simulink model "FMReceiverSimulinkExample"  (R2022b)
settings: Solver=FixedStepDiscrete  StartTime=0.0  StopTime=inf  RelTol=1e-3
PreLoadFcn:
  | fmRxParams = helperFMConfig;
PostLoadFcn:
  | rxBlock = find_system(gcs, 'MaskType', 'SDRu Receiver');
  | if exist('sdruroot', 'file')
  |     setupsdru;
  |     connectedRadios = findsdru;
  |     if strncmp(connectedRadios(1).Status, 'Success', 7)
  |         platform = connectedRadios(1).Platform;
  |         set_param(rxBlock{1}, 'Platform', platform);
  |         switch connectedRadios(1).Platform
  |             case {'B200','B210'}
  |                 address = connectedRadios(1).SerialNum;
  |                 fmRxParams.MasterClockRate = 20e6;
  |                 fmRxParams.DecimationFactor = (fmRxParams.MasterClockRate)/200e3;
  | %                 set_param(rxBlock{1}, 'masterClkRateB210', 'fmRxParams.MasterClockRate');
  | %                 set_param(rxBlock{1}, 'masterClkRateB200', 'fmRxParams.MasterClockRate');
  | %                 set_param(rxBlock{1}, 'decimInterp', 'fmRxParams.DecimationFactor');
  |             case {'X300','X310','N320/N321'}
  |                 address = connectedRadios(1).IPAddress;
  |                 fmRxParams.MasterClockRate = 200e6;
  |                 fmRxParams.DecimationFactor = (fmRxParams.MasterClockRate)/200e3;
  |             case {'N300','N310'}
  |                 address = connectedRadios(1).IPAddress;
  |                 fmRxParams.MasterClockRate = 153.6e6;
  |                 fmRxParams.DecimationFactor = (fmRxParams.MasterClockRate)/200e3;
  |             case {'N200/N210/USRP2'}
  |                 address = connectedRadios(1).IPAddress;
  |                 fmRxParams.MasterClockRate = 100e6;
  |                 fmRxParams.DecimationFactor = (fmRxParams.MasterClockRate)/200e3;
  |         end
  |     else
  |         platform = 'N200/N210/USRP2';
  |         address = '192.168.10.2';
  |         set_param(rxBlock{1}, 'Platform', platform);
  |         fmRxParams.MasterClockRate = 100e6;
  |         fmRxParams.DecimationFactor = (fmRxParams.MasterClockRate)/200e3;
  |     end
  |     set_param(rxBlock{1}, 'USRP_ID', address);
  | end
InitFcn:
  | fmRxParams = helperFMConfig;
  | 
  | if (strcmp(get_param([gcs '/Signal Source Selector'],'OverrideUsingVariant'),'V_4'))
  | rxBlock = find_system(gcs, 'MaskType', 'SDRu Receiver');
  | platform = get_param(rxBlock{1}, 'platform');
  | 
  | switch platform
  |     case {'B200','B210'}
  |         fmRxParams.MasterClockRate = 20e6;
  |         fmRxParams.DecimationFactor = (fmRxParams.MasterClockRate)/200e3;
  |     case {'X300','X310','N320/N321'}
  |         fmRxParams.MasterClockRate = 200e6;
  |         fmRxParams.DecimationFactor = (fmRxParams.MasterClockRate)/200e3;
  |     case {'N300','N310'}
  |         fmRxParams.MasterClockRate = 153.6e6;
  |         fmRxParams.DecimationFactor = (fmRxParams.MasterClockRate)/200e3;
  |     case {'N200/N210/USRP2'}
  |         fmRxParams.MasterClockRate = 100e6;
  |         fmRxParams.DecimationFactor = (fmRxParams.MasterClockRate)/200e3;
  | end
  | end
  | % fmRxParams = helperFMConfig;
  | % rxBlocks = find_system(gcs, 'MaskType', 'SDRu Receiver');
  | % block = rxBlocks{1};
  | % platform = get_param(block, 'platform');
  | % fmRxParams.Gain = evalin('base', get_param(block,'Gain'));
  | % fmRxParams.DecimationFactor = evalin('base', get_param(block,'decimInterp'));
  | % switch platform
  | %     case 'B200'
  | %         fmRxParams.MasterClockRate = evalin('base', get_param(block,'masterClkRateB200'));
  | %     case 'B210'
  | %         fmRxParams.MasterClockRate = evalin('base', get_param(block,'masterClkRateB210'));
  | %     case 'X300'
  | %         if strcmp(get_param(block,'IsTwinRXDaughterboard'),'on')
  | %             fmRxParams.MasterClockRate = evalin('base', get_param(block,'masterClkRateTwinRX'));
  | %         else
  | %             fmRxParams.MasterClockRate = evalin('base', get_param(block,'masterClkRateX300'));
  | %         end
  | %     case 'X310'
  | %         if strcmp(get_param(block,'IsTwinRXDaughterboard'),'on')
  | %             fmRxParams.MasterClockRate = evalin('base', get_param(block,'masterClkRateTwinRX'));
  | %         else
  | %             fmRxParams.MasterClockRate = evalin('base', get_param(block,'masterClkRateX310'));
  | %         end
  | %     case 'N300'
  | %         fmRxParams.MasterClockRate = evalin('base', get_param(block,'masterClkRateN300'));
  | %     case 'N310'
  | %         fmRxParams.MasterClockRate = evalin('base', get_param(block,'masterClkRateN310'));
  | %     case 'N320/N321'
  | %         fmRxParams.MasterClockRate = evalin('base', get_param(block,'masterClkRateN320'));
  | %     otherwise
  | %         fmRxParams.MasterClockRate = evalin('base', get_param(block,'masterClkRate'));
  | % end
undefined symbols (not defined in the file or in its folder): Fs, ip, usb
libraries: simulink x2, plutoradiolib x1, dspsnks4 x1, commsource2 x1, commanabbnd3 x1, sdrrlib x1, commsdrhw_v2 x1
Description:
  | This model uses either captured signals, or receive signals in real time
  | using RTL-SDR radio, ADALM-PLUTO radio or USRP radio with Simulink(R) to perform FM
  | demodulation and mono decoding.
settings Model: Creator=The MathWorks, Inc.  LastModifiedBy=The MathWorks, Inc.
settings SolverCC: AlgebraicLoopSolver=TrustRegion  MaxZcPerStep=1
settings DataIOCC: SaveFormat=Structure  SaveOutput=off  SignalLogging=off  DSMLogging=off  SaveTime=off  ReturnWorkspaceOutputs=off
settings OptimizationCC: ExpressionDepthLimit=2147483647  EfficientMapNaN2IntZero=off  LifeSpan=inf  SimCompilerOptimization=on
settings DebuggingCC: UnderspecifiedInitializationDetection=Classic  MergeDetectMultiDrivingBlocksExec=none  SolverPrmCheckMsg=warning  InheritedTsInSrcMsg=none  MultiTaskCondExecSysMsg=none  ParameterPrecisionLossMsg=none  FcnCallInpInsideContextMsg=warning  UnconnectedInputMsg=warning  UnconnectedOutputMsg=warning  UnconnectedLineMsg=warning  AllowSymbolicDim=off  StateNameClashWarn=warning  SFUnexpectedBacktrackingDiag=warning  SFNoUnconditionalDefaultTransitionDiag=warning  SFExecutionAtInitializationDiag=none  SFMachineParentedDataDiag=warning  ArithmeticOperatorsInVariantConditions=warning
settings HardwareCC: ProdBitPerPointer=32  ProdBitPerSizeT=32  ProdBitPerPtrDiffT=32  ProdLargestAtomicFloat=None  ProdIntDivRoundTo=Undefined  ProdEndianess=Unspecified  ProdWordSize=32  ProdHWDeviceType=32-bit Generic  TargetBitPerLong=64  TargetBitPerPointer=64  TargetBitPerSizeT=64  TargetBitPerPtrDiffT=64  TargetLongLongMode=on  TargetIntDivRoundTo=Zero  TargetEndianess=LittleEndian  TargetWordSize=64  TargetHWDeviceType=Generic->MATLAB Host Computer  ProdEqTarget=off
settings ModelReferenceCC: EnableRefExpFcnMdlSchedulingChecks=on  PropagateSignalLabelsOutOfModel=off
settings SFSimCC: SimIntegrity=off  SimUseLocalCustomCode=off  CustomCodeUndefinedFunction=UseInterfaceOnly
settings RTWCC: RTWUseLocalCustomCode=off
settings RTWCC: CustomSourceCode=|
  | #include <stdio.h>
  | #include <stdlib.h>
settings CodeAppCC: MaxIdLength=128  StateflowObjectComments=on
settings GRTTargetCC: TargetLangStandard=C89/C90 (ANSI)  CombineOutputUpdateFcns=off  GRTInterface=on
settings ConfigComp: CovMetricSettings=dw  CovSaveCumulativeToWorkspaceVar=on  CovSaveSingleToWorkspaceVar=on  CovExternalEMLEnable=off  CovSFcnEnable=off

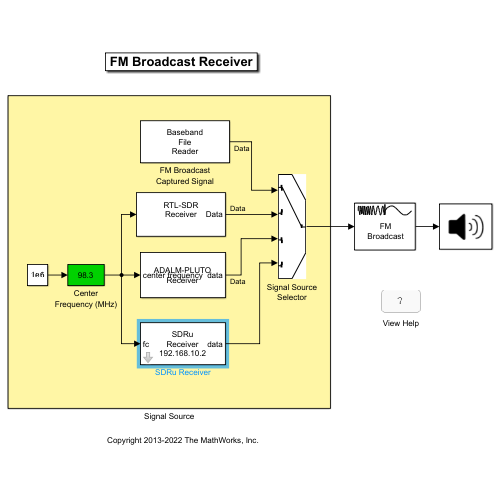
[thumbnail: Simulink's stored preview of the top-level diagram]
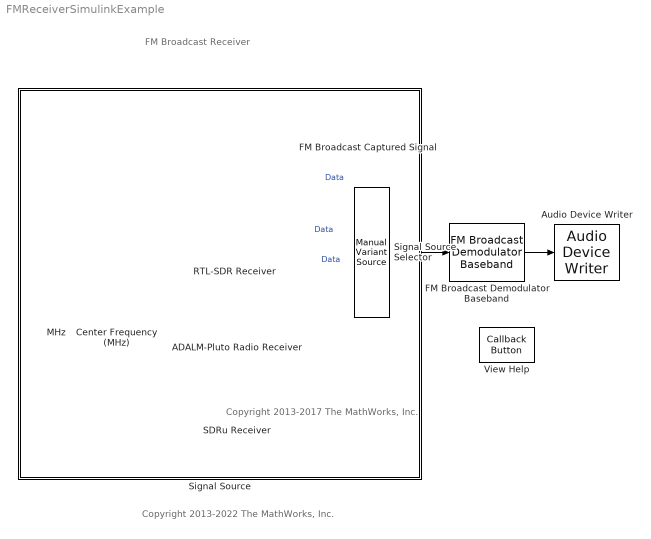
== system FMReceiverSimulinkExample ==
  note: FM Broadcast Receiver
  note: Copyright 2013-2017 The MathWorks, Inc.
  note: Copyright 2013-2022 The MathWorks, Inc.
  ADALM-Pluto Radio Receiver : plutoradiolib/ADALM-Pluto Radio Receiver  RadioID=usb:0  uri=ip:10.0.0.200  CenterFrequencySource=Input Port  CenterFrequency=2.4e9  GainSource=AGC Slow Attack  GainSourceBlock=AGC Slow Attack  Gain=10  ChannelMapping=1  BasebandSampleRate=fmRxParams.FrontEndSampleRate  OutputDataType=single  SamplesPerFrame=fmRxParams.FrontEndSamplesPerFrame  OverflowOutputPort=off  EnableBurstMode=off  NumFramesInBurst=1  ShowAdvancedProperties=off  UseCustomFilter=off  filtPathRates=[ 737280000, 11520000, 3840000, 1920000, 960000, 240000 ]  filtCoefficients=round( fir1( 127, 0.75 )*2^15*10^1.2 )  filtCoefficientSize=128  filtDecimInterpFactor=4  filtGain=-12  filtRFBandwidth=18e6  filterConfigStruct=struct()  EnableQuadratureCorrection=on  EnableRFDCCorrection=on  EnableBasebandDCCorrection=on  FrequencyCorrection=0  OverrideSampleTime=off  SampleTime=0.02  DataTimeout=Inf  ENSMPinControlMode=None  BISTLoopbackMode=Disabled  BISTToneInject=Disabled  BISTSignalGen=PRBS  BISTToneFreq=Fs/32  BISTToneLevel=0
  Audio Device Writer : dspsnks4/Audio Device Writer  Driver=ALSA  Device=Default  InheritSampleRate=on  SampleRate=44100  BitDepth=16-bit integer  BufferSize=4096  NumBuffers=10  DefaultOutputChannelMapping=on  OutputChannelMapping=1:2  OutputNumUnderrunSamples=off  DriverIdx=8  DeviceWarnFlag=''
  Center Frequency (MHz) : simulink/Math Operations/Slider Gain  gain=98.3  low=87.9  high=107.9
  FM Broadcast Captured Signal : commsource2/Baseband File Reader  Filename=rbds_capture.bb  InheritSampleTimeFromFile=on  SampleTime=1  SamplesPerFrame=fmRxParams.FrontEndSamplesPerFrame  CyclicRepetition=on  FileEndOutputPort=off  SimulateUsing=Code generation
  FM Broadcast Demodulator Baseband : commanabbnd3/FM Broadcast Demodulator Baseband  SampleRate=fmRxParams.FrontEndSampleRate  FrequencyDeviation=fmRxParams.FrequencyDeviation  FilterTimeConstant=fmRxParams.FilterTimeConstant  AudioSampleRate=fmRxParams.AudioSampleRate  PlaySound=off  BufferSize=fmRxParams.BufferSize  Stereo=off  RBDS=off  RBDSSamplesPerSymbol=10  RBDSCostasLoop=off  SimulateUsing=Code generation
  MHz : Constant  Value=1e6  VectorParams1D=off  SampleTime=-1  FramePeriod=-1
  RTL-SDR Receiver : sdrrlib/RTL-SDR Receiver  IPAddress=0  CenterFrequencySource=Input port  CenterFrequency=102.5e6  GainSource=AGC  Gain=0  ADCRate=fmRxParams.FrontEndSampleRate  FrequencyCorrection=0  LostSamplesOutputPort=off  LatencyOutputPort=off  OutputDataType=single  FrameLength=fmRxParams.FrontEndSamplesPerFrame  EnableBurstMode=off  NumFramesInBurst=20  sobjType=sdrr.internal.SDRRTLReceiverSL  dataUDPPort=-1  ctrlUDPPort=-1  subDeviceList=nosubdev  sdrBlockType=SDRBlockTypeSLT.SDRRxBlock  requester=UNUSED_BY_SFCN  sdrExecutionMode=SDRExecutionModeSLT.ExecModeHW  BypassUserLogic=off  DecimatorSelect=DDC decimator  SourceSelect=RF data  SineAmplitude=16000  EnableInternalClock=off  BypassIQBalance=off  IFBandwidth=40e6  ADCRateSource=Dialog  IntermediateFrequency=0  DecimationFactorSource=Dialog  DecimationFactor=512  RFFrequencyIsTunable=logical(1)  SampleTime=(fmRxParams.FrontEndSamplesPerFrame)/(fmRxParams.FrontEndSampleRate)  IFBandwidthSource=Dialog  SineFrequency=30000  BypassDCBlockingFilter=off  IntermediateFrequencySource=Dialog  IQBalanceCoefficients=64  SkipAllHardwareResetAndInitialization=off  EnableIQCalibrationTable=on  CacheIQCalibrationTable=off  EnableOffsetTuning=off  EnableRTLAGC=off  EnableTestMode=off  EnableTunerAGC=on  FrequencyCorrectionSource=Dialog  NumMLBuffers=128  NumUSBBuffers=16  RTLCrystalFrequency=28800000  TunerCrystalFrequency=28800000
  SDRu Receiver : commsdrhw_v2/SDRu Receiver  rxtx=rx  initializeIPAddress=0  devMap=10  USRP2_IP=192.168.10.2  USRP_IP_X300=192.168.10.2  USRP_IP_X310=No devices found  USRP_IP_N300=192.168.10.2  USRP_IP_N310=192.168.10.2  USRP_IP_N320=192.168.20.2  USRP_serialNumB200=30EA06C  USRP_serialNumB210=30F597A  platform=N200/N210/USRP2  prevPlatform=B200  lastIPAddressPopup=192.168.10.2  USRP_ID=192.168.10.2  LastIPAddress=192.168.10.2  IsTwinRXDaughterboard=off  EnableTwinRXPhaseSync=off  losrc=0  ChannelMapping=1  centerFrequencySrc=Input port  centerFrequency=2.45e9  loOffsetSrc=Dialog  loOffset=0  gainSrc=Dialog  gain=fmRxParams.Gain  PPSSource=Internal  EnableGPSLock=off  EnsureSyncGPSTime=off  clockSource=Internal  EnableRefLock=off  masterClkRateParam=100e6  masterClkRateB200=fmRxParams.MasterClockRate  masterClkRateB210=fmRxParams.MasterClockRate  masterClkRateX300=200e6  masterClkRateX310=200e6  masterClkRateN300=125e6  masterClkRateN310=125e6  masterClkRateN320=200e6  masterClkRate=100e6  masterClkRateTwinRX=200e6  decimInterpSrc=Dialog  decimInterpPort=512  lastDecimSource=Dialog  decimInterp=fmRxParams.DecimationFactor  USRP2_IP_NUM=[49 57 50 46 49 54 56 46 49 48 46 50]  sampleRate=200000  sampleTime=(500)/100000000  TransportDataType=int16  overrunUnderrunPort=off  dataLengthPort=off  EnableTimeStamps=off  outputDatatype=single  frameLength=fmRxParams.FrontEndSamplesPerFrame  HOST_DATA_PORT=0  HOST_CONTROL_PORT=0  USRP2_DATA_PORT=0  USRP2_CONTROL_PORT=0  bufferMode=Continuous streaming  EnableBurstMode=off  NumFramesInBurst=100
  Signal Source : Subsystem
      mask Display: disp('')
  Signal Source Selector : simulink/Signal Routing/Manual Variant Source  NumChoices=4  LabelModeActiveChoice=V_1
  View Help : CallbackButton  ButtonText=?
      settings: ClickFcn=showExample('comm/FMBroadcastReceiverInSimulinkExample')
  wires:
  ADALM-Pluto Radio Receiver/1 -> Signal Source Selector/3  "Data"
  FM Broadcast Captured Signal/1 -> Signal Source Selector/1  "Data"
  FM Broadcast Demodulator Baseband/1 -> Audio Device Writer/1
  SDRu Receiver/1 -> Signal Source Selector/4
  RTL-SDR Receiver/1 -> Signal Source Selector/2  "Data"
  Center Frequency (MHz)/1 -> RTL-SDR Receiver/1, SDRu Receiver/1, ADALM-Pluto Radio Receiver/1
  MHz/1 -> Center Frequency (MHz)/1
  Signal Source Selector/1 -> FM Broadcast Demodulator Baseband/1

== system FMReceiverSimulinkExample/Signal Source ==
